simulink model "tanhsim"  (R2020a)
settings: Solver=VariableStepAuto  StartTime=0.0  StopTime=10.0  RelTol=1e-3
undefined symbols (not defined in the file): x1
settings Model: Creator=Mahsa  LastModifiedBy=Mahsa

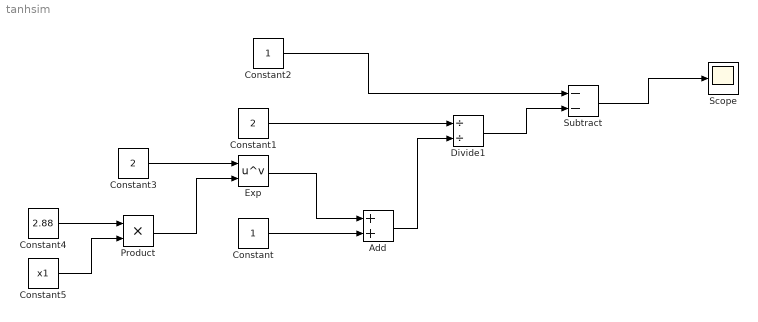
== system tanhsim ==
  Add : Sum
  Constant : Constant
  Constant1 : Constant  Value=2
  Constant2 : Constant
  Constant3 : Constant  Value=2  OutDataTypeStr=double
  Constant4 : Constant  Value=2.88  OutDataTypeStr=double
  Constant5 : Constant  Value=x1  VectorParams1D=off  OutMin=-4  OutMax=4
  Divide1 : Product  Inputs=//
  Exp : Math  Operator=pow  OutMin=-1  OutMax=1  SaturateOnIntegerOverflow=on
  Product : Product
  Scope : Scope
  Subtract : Sum  Inputs=--
  wires:
  Constant/1 -> Add/2
  Constant1/1 -> Divide1/1
  Exp/1 -> Add/1
  Constant2/1 -> Subtract/1
  Add/1 -> Divide1/2
  Constant3/1 -> Exp/1
  Constant4/1 -> Product/1
  Constant5/1 -> Product/2
  Product/1 -> Exp/2
  Divide1/1 -> Subtract/2
  Subtract/1 -> Scope/1
